simulink model "UIF_LED_ColorCode"  (R2022b)
settings: Solver=FixedStepDiscrete  StartTime=0.0  StopTime=10.0  RelTol=1e-3  EnableMultiTasking=on
InitFcn:
  | mbd_mpc_consistency_checks(bdroot(gcs));
undefined symbols (not defined in the file): LQFP
libraries: mbd_mpc574x_ec_toolbox x4, simulink x4
settings Model: Creator=MAAM  LastModifiedBy=MAAM
settings DataIOCC: ExternalInput=off  InitialState=off  SaveOutput=off  SignalLogging=off  SaveTime=off
settings OptimizationCC: DefaultParameterBehavior=Inlined  EnhancedBackFolding=on  PassReuseOutputArgsAs=Individual arguments  ZeroExternalMemoryAtStartup=off  ZeroInternalMemoryAtStartup=off  OptimizeBlockOrder=speed  DifferentSizesBufferReuse=on  OptimizationCustomize=off  EfficientTunableParamExpr=on
settings DebuggingCC: InheritedTsInSrcMsg=none  ParameterTunabilityLossMsg=error
settings HardwareCC: ProdBitPerPointer=32  ProdBitPerSizeT=32  ProdBitPerPtrDiffT=32  ProdLargestAtomicInteger=Long  ProdLargestAtomicFloat=Double  ProdEndianess=BigEndian  ProdWordSize=32  ProdHWDeviceType=Motorola PowerPC
settings SFSimCC: MATLABDynamicMemAlloc=off
settings RTWCC: Description=Model Based Design Toolbox MPC57xx Code Generation Target  SystemTargetFile=mbd_mpc574x.tlc  MakeCommand=mbd_mpc574x_make_rtw  TemplateMakefile=mbd_mpc574x.tmf
settings CodeAppCC: ForceParamTrailComments=on  IgnoreCustomStorageClasses=off  OperatorAnnotations=on  SimulinkDataObjDesc=on  SFDataObjDesc=on  InsertBlockDesc=on
settings STFCustomTargetCC: TargetLangStandard=C99 (ISO)  MultiwordLength=256  CombineOutputUpdateFcns=on  ERTCustomFileBanners=on  SupportContinuousTime=off  SupportNonInlinedSFcns=off  RemoveResetFunc=on  MATLABClassNameForMDSCustomization=Simulink.SoftwareTarget.ERTCustomization  SystemTargetFile=mbd_mpc574x.tlc
settings ERTTargetCC: TargetLangStandard=C99 (ISO)  ParMdlRefBuildCompliant=off  CompOptLevelCompliant=off  ConcurrentExecutionCompliant=off  ModelStepFunctionPrototypeControlCompliant=off  CPPClassGenCompliant=off  UseToolchainInfoCompliant=off  InlinedParameterPlacement=NonHierarchical  ERTCustomFileTemplate=example_file_process.tlc

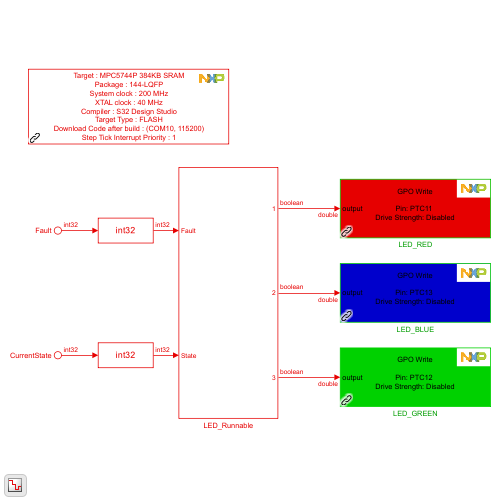
[thumbnail: Simulink's stored preview of the top-level diagram]
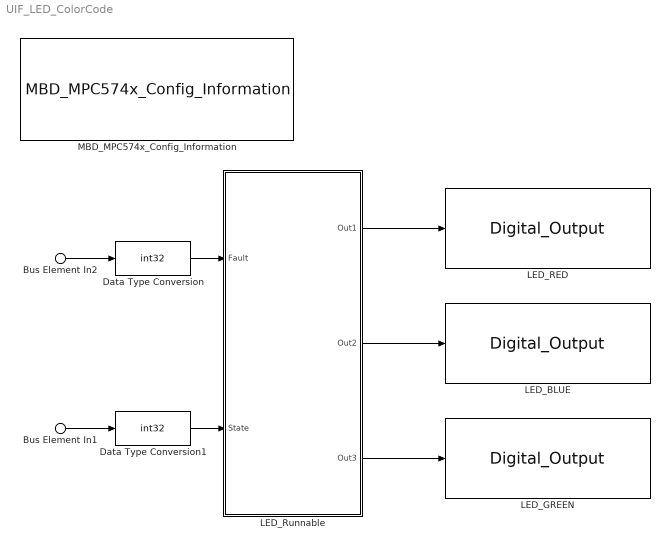
== system UIF_LED_ColorCode ==
  Bus Element In1 : Inport  PortName=CurrentState
  Bus Element In2 : Inport  Port=2  PortName=Fault
  Data Type Conversion : DataTypeConversion  OutDataTypeStr=int32  SaturateOnIntegerOverflow=off  RndMeth=Floor
  Data Type Conversion1 : DataTypeConversion  OutDataTypeStr=int32  SaturateOnIntegerOverflow=off  RndMeth=Floor
  LED_BLUE : mbd_mpc574x_ec_toolbox/GPIO Blocks/Digital_Output  gpio_pin=PTC13: [SIUL2_GPIO45 | General Purpose IO PC[13]]  gpio_drive_strength=Disabled
  LED_GREEN : mbd_mpc574x_ec_toolbox/GPIO Blocks/Digital_Output  gpio_pin=PTC12: [SIUL2_GPIO44 | General Purpose IO PC[12]]  gpio_drive_strength=Disabled
  LED_RED : mbd_mpc574x_ec_toolbox/GPIO Blocks/Digital_Output  gpio_pin=PTC11: [SIUL2_GPIO43 | General Purpose IO PC[11]]  gpio_drive_strength=Disabled
  LED_Runnable : Subsystem
  MBD_MPC574x_Config_Information : mbd_mpc574x_ec_toolbox/MBD_MPC574x_Config_Information  Priority=1  disp_str=|  config_params=[]  mcu_target_name=MPC5744P  mcu_target_package=144-LQFP  mcu_target_sram_size=384KB  mcu_system_clock_freq=200  mcu_xtal_freq=40  mcu_step_timer=PIT Channel 0  mcu_step_priority=1  ds_import_enable=on  target_compiler=S32 Design Studio  target_memory=FLASH  s32ds_target_compile_opts=-g3 -mbig -mvle -O1 -mregnames -mlsp -specs=ewl_c9x.specs -mhard-float -Wall -c -std=c99 -fdata-sections -ffunction-sections -funsigned-char -fmessage-length=0 -nostdinc -fno-jump-tables -DTURN_ON_CPU0  s32ds_target_assemble_opts=-g3 -mbig -mvle -mregnames -O1 -DTURN_ON_CPU0 -mhard-float  s32ds_target_link_opts=-Xlinker -gc-sections  s32ds_target_default_lcf=on  s32ds_target_user_lcf=MPC5744P_flash.ld  ghs_target_compile_opts=-G -filetype.c  ghs_target_assemble_opts=-G -filetype.assembly  ghs_target_default_lcf=on  ghs_target_user_lcf=MPC5744P_flash.ld  diab_target_compile_opts=-@E+err.log -c -g -Xenum-is-best -Xlint -Xnested-interrupts -Xdebug-local-cie -Xclib-optim-off -Xc-new  diab_target_assemble_opts=-@E+err.log -l -g  diab_target_link_opts=-@E+err.log -Ws -m6 -lc -lm  diab_target_default_lcf=on  diab_target_user_lcf=MPC5744P_flash.dld  pil_download_enable=off  rbl_download_enable=on  rbl_start_delay=5000  rbl_restart_request=on  rbl_com_port=Custom  rbl_com_port_custom=COM10  pil_download_rate=115200  pil_interface=Serial 0  pil_rx=PTB3: [LIN0_RX | LIN 0 Receive Pin]  pil_tx=PTB2: [LIN0_TX | LINFlexD 0 Transmit Pin]  rbl_def_password=on  rbl_password=0xFEEDFACECAFEBEEF  rbl_manual_len_size=off  rbl_start_address=0  rbl_code_size=0  ADC_PcrCheckEnDis=on  FlexPWM_PcrCheckEnDis=on  CTU_PcrCheckEnDis=on  SWG_PcrCheckEnDis=on  eTimer_PcrCheckEnDis=off  EQADC_PcrCheckEnDis=on  eMIOS_PcrCheckEnDis=on  FlexCAN_PcrCheckEnDis=on  I2C_PcrCheckEnDis=on  MCAN_PcrCheckEnDis=on  SPI_PcrCheckEnDis=on  UART_PcrCheckEnDis=on  GPIO_OutputPcrCheckEnDis=on  GPIO_InputPcrCheckEnDis=on  eDMA_PcrCheckEnDis=on  PIT_PcrCheckEnDis=on  AMMCLIB_PcrCheckEnDis=on  FM_PcrCheckEnDis=on  Profiler_PcrCheckEnDis=on  ModelRef_PcrCheckEnDis=on  ModelPinCheck_PcrCheckEnDis=on
      | System Clock : 200 MHz
      | Target : MPC5744P
      | Package : 144LQFP
      | XTAL Freq : 40 MHz
      | Compiler : S32 Design Studio
      | Target Type : FLASH
      | Global Interrupt Priority : 8
      | System Tick Interrupt Priority : 12
      | Freemaster : None;
      | Download Code after build : off
  wires:
  Data Type Conversion1/1 -> LED_Runnable/2(State)
  Data Type Conversion/1 -> LED_Runnable/1(Fault)
  LED_Runnable/3(Out3) -> LED_GREEN/1
  LED_Runnable/2(Out2) -> LED_BLUE/1
  LED_Runnable/1(Out1) -> LED_RED/1
  Bus Element In2/1 -> Data Type Conversion/1
  Bus Element In1/1 -> Data Type Conversion1/1

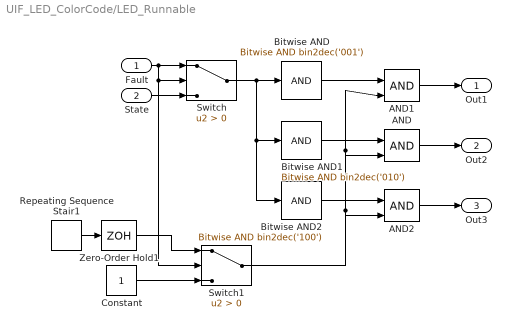
== system UIF_LED_ColorCode/LED_Runnable ==
  Fault : Inport
  State : Inport  Port=2
  AND : Logic  IconShape=distinctive  AllPortsSameDT=off  OutDataTypeStr=boolean
  AND1 : Logic  IconShape=distinctive  AllPortsSameDT=off  OutDataTypeStr=boolean
  AND2 : Logic  IconShape=distinctive  AllPortsSameDT=off  OutDataTypeStr=boolean
  Bitwise AND : simulink/Logic and Bit Operations/Bitwise Operator  logicop=AND  UseBitMask=on  BitMask=bin2dec('001')  BitMaskRealWorld=Stored Integer
      settings: LibrarySourceBlock=|
      | simulink/Quick Insert/Logic and Bit
      | Operations/Bitwise AND
  Bitwise AND1 : simulink/Logic and Bit Operations/Bitwise Operator  logicop=AND  UseBitMask=on  BitMask=bin2dec('010')  BitMaskRealWorld=Stored Integer
      settings: LibrarySourceBlock=|
      | simulink/Quick Insert/Logic and Bit
      | Operations/Bitwise AND
  Bitwise AND2 : simulink/Logic and Bit Operations/Bitwise Operator  logicop=AND  UseBitMask=on  BitMask=bin2dec('100')  BitMaskRealWorld=Stored Integer
      settings: LibrarySourceBlock=|
      | simulink/Quick Insert/Logic and Bit
      | Operations/Bitwise AND
  Constant : Constant
  Repeating Sequence Stair1 : simulink/Sources/Repeating Sequence Stair  OutValues=[0 1].'  tsamp=-1  OutMin=[]  OutMax=[]  OutDataTypeStr=double  OutputDataTypeScalingMode=double  OutDataType=fixdt(0,8)  ConRadixGroup=Best Precision: Vector-wise  OutScaling=2^-12
  Switch : Switch  Criteria=u2 > Threshold  SaturateOnIntegerOverflow=off  InputSameDT=off
  Switch1 : Switch  Criteria=u2 > Threshold  SaturateOnIntegerOverflow=off  InputSameDT=off
  Zero-Order Hold1 : ZeroOrderHold  SampleTime=0.1
  Out1 : Outport
  Out2 : Outport  Port=2
  Out3 : Outport  Port=3
  wires:
  Bitwise AND1/1 -> AND/1
  Switch1/1 -> AND2/2, AND1/2, AND/2
  Switch/1 -> Bitwise AND/1, Bitwise AND1/1, Bitwise AND2/1
  Fault/1 -> Switch/1, Switch/2, Switch1/2
  Repeating Sequence Stair1/1 -> Zero-Order Hold1/1
  AND2/1 -> Out3/1
  AND1/1 -> Out1/1
  State/1 -> Switch/3
  Constant/1 -> Switch1/3
  AND/1 -> Out2/1
  Bitwise AND/1 -> AND1/1
  Bitwise AND2/1 -> AND2/1
  Zero-Order Hold1/1 -> Switch1/1
